simulink model "NMPC_UAV_MHE_CasaDi"  (R2022a)
settings: Solver=VariableStepAuto  StartTime=0.0  StopTime=60*2  RelTol=1e-3
values from neighbouring files (symbols this model uses):
  g = [g; st_next-st_next_RK4]    [MHE_CasaDi.m]    (also in UAVStateJacobianFcn.m = 9.81; UAV_parameters.m = 9.81)
  mass = 0.5    [MHE_CasaDi.m]    (also in UAV_parameters.m)
  Optitrack_Ts = 1/120    (= 0.00833333333333)    [Optitrack_parameters.m]
  Optitrack_var = [0.02e-3; 0.02e-3; 0.02e-3; 0.1*pi/180; 0.1*pi/180; 0.1*pi/180]    [Optitrack_parameters.m]
  Ts = 0.1    [MHE_CasaDi.m]    (also in UAV_parameters.m)
  XYThetaVPred = [1.99999737442 0.0050155230369 1.57305810416 0.100033273961 1.99990290242 0.0193669877756 1.58175256385 0.186831373139 1.99953586241 0.0406259992754 1.59458893555 0.23874169648 ... (4804 elements, 4x1201)]    [XYThetaVPred_wObstacles.mat]
  ZRef = 2*ones(1,60*2*10+1)    [UAV_parameters.m]
libraries: mpclib x1
settings Model: Creator=mrnel  LastModifiedBy=root

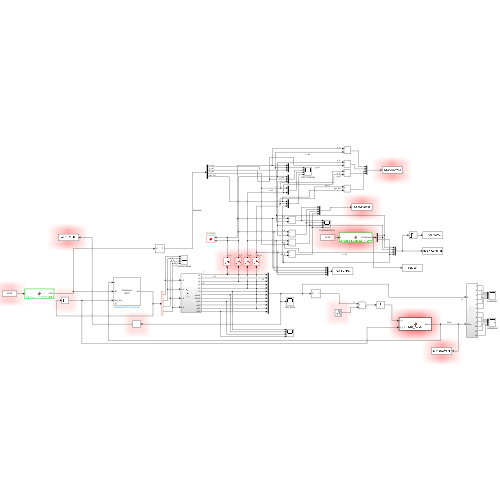
[thumbnail: Simulink's stored preview of the top-level diagram]
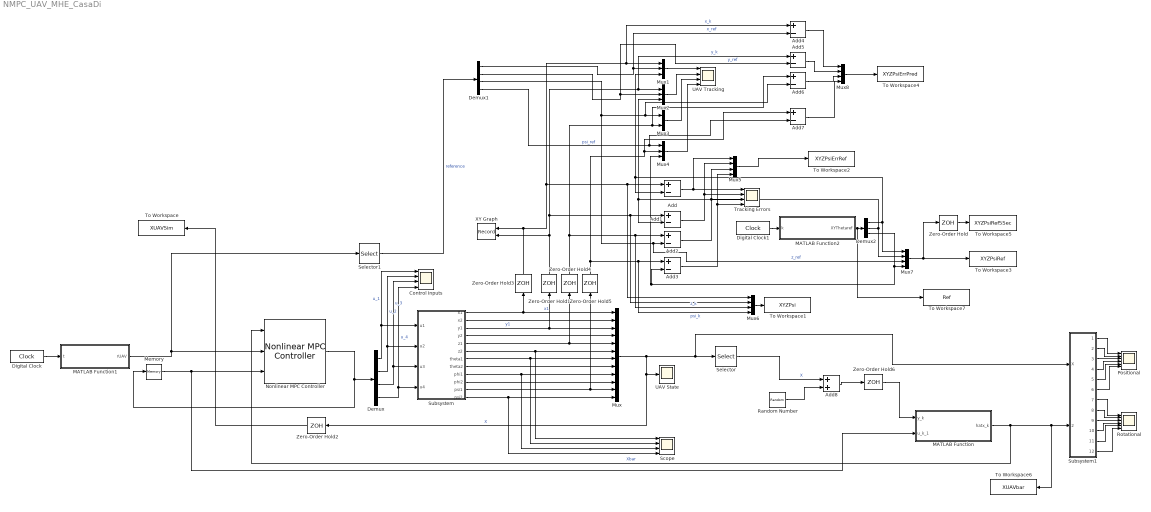
== system NMPC_UAV_MHE_CasaDi ==
  Add{,1..7} (8 alike) : Sum  Inputs=+-
  Add8 : Sum
  Control Inputs : Scope  NumInputPorts=4
  Demux : Demux
  Demux1 : Demux
  Demux2 : Demux  Outputs=3
  Digital Clock : DigitalClock  SampleTime=Ts
  Digital Clock1 : DigitalClock  SampleTime=Ts
  MATLAB Function : MATLAB Function  TreatAsAtomicUnit=on  SystemSampleTime=Ts
  MATLAB Function1 : MATLAB Function  TreatAsAtomicUnit=on
  MATLAB Function2 : MATLAB Function  TreatAsAtomicUnit=on  SystemSampleTime=Ts
  Memory : Memory  InitialCondition=[mass*g;0;0;0]  InheritSampleTime=on
  Mux : Mux  Inputs=12
  Mux1 : Mux  Inputs=3
  Mux2 : Mux  Inputs=3
  Mux3 : Mux  Inputs=2
  Mux4 : Mux  Inputs=3
  Mux{5..8} (4 alike) : Mux
  Nonlinear MPC Controller : mpclib/Nonlinear MPC Controller  nlmpcobj=nlmpcobj  UseObjectTs=on  UseMEX=off  md_enabled=off  mvtarget_enabled=off  param_enabled=off  cost_enabled=off  mvseq_enabled=off  stateseq_enabled=off  ovseq_enabled=off  slack_enabled=off  status_enabled=off  ov_min=off  ov_max=off  mv_min=off  mv_max=off  mvrate_min=off  mvrate_max=off  state_min=off  state_max=off  ov_weight=off  mv_weight=off  mvrate_weight=off  ecr_weight=off  nlp_initialize=off
  "Positional " : Scope  NumInputPorts=6
  Random Number : RandomNumber  Mean=zeros(6,1)  Variance=Optitrack_var.^2  SampleTime=Optitrack_Ts
  Rotational : Scope  NumInputPorts=6
  Scope : Scope  NumInputPorts=4
  Selector : Selector  NumberOfDimensions=2  InputPortWidth=3  IndexOptions=Index vector (dialog),Index vector (dialog)  Indices=[1 3 5 7 9 11],1  OutputSizes=1,1
  Selector1 : Selector  NumberOfDimensions=2  InputPortWidth=3  IndexOptions=Index vector (dialog),Index vector (dialog)  Indices=1,[1 3 5 11]  OutputSizes=1,1
  Subsystem : Subsystem
  Subsystem1 : Subsystem
  To Workspace : ToWorkspace  VariableName=XUAVSim  SaveFormat=Timeseries  SampleTime=Ts
  To Workspace1 : ToWorkspace  VariableName=XYZPsi  SaveFormat=Timeseries  SampleTime=0.1
  To Workspace2 : ToWorkspace  VariableName=XYZPsiErrRef  SaveFormat=Timeseries  SampleTime=Ts
  To Workspace3 : ToWorkspace  VariableName=XYZPsiRef  SaveFormat=Timeseries  SampleTime=0.1
  To Workspace4 : ToWorkspace  VariableName=XYZPsiErrPred  SaveFormat=Timeseries  SampleTime=Ts
  To Workspace5 : ToWorkspace  VariableName=XYZPsiRef5Sec  SaveFormat=Timeseries  SampleTime=5
  To Workspace6 : ToWorkspace  VariableName=XUAVbar  SaveFormat=Timeseries  SampleTime=Ts
  To Workspace7 : ToWorkspace  VariableName=Ref  SaveFormat=Timeseries  SampleTime=-1
  Tracking Errors : Scope  NumInputPorts=4
  UAV State : Scope
  UAV Tracking : Scope  NumInputPorts=4
  XY Graph : Record  FileSettingsInternal="{\"entries\":[{\"content\":{\"excelSettings\":{\"content\":{},\"type\":\"Streamout.ExcelSettings\"}},\"type\":\"Streamout.FileSettingStorage\",\"uuid\":\"\"}],\"packageUris\":[\"http:\\/\\/schema.mathworks.com\\/mf0\\/streamout_blocks\\/R2020a\"],\"version\":\"1.0\"}"  Layout=[1 1]  SignalsInternal="{\"entries\":[{\"content\":{\"signals\":[{\"content\":{\"blockPath\":[],\"channel\":[],\"dimensions\":[1],\"domain\":\"\",\"lineColor\":\"#a2142f\",\"plots\":[1],\"port\":1,\"sid\":[],\"signalID\":495,\"signalName\":\"x_k\"},\"type\":\"RecordBlkView.Signal\",\"uuid\":\"\"},{\"content\":{\"blockPath\":[],\"channel\":[],\"dimensions\":[1],\"domain\":\"\",\"lineColor\":\"#139fff\",\"plots\":[1],\"port\":2,\"sid\":[],\"signalID\":498,\"signalName\":\"y_k\"},\"type\":\"RecordBlkView.Signal\",\"uuid\":\"\"}]},\"type\":\"RecordBlkView.InputSignals\",\"uuid\":\"\"}],\"packageUris\":[\"http:\\/\\/schema.mathworks.com\\/mf0\\/streamout_blocks\\/R2020a\"],\"version\":\"1.0\"}"  VisualizationBindings="{\"xyplotplugin\":{\"info\":[{\"series\":[{\"bindingParametersList\":[{\"parameter\":\"X-Axis\",\"signalID\":495,\"signalName\":\"x_k\"},{\"parameter\":\"Y-Axis\",\"signalID\":498,\"signalName\":\"y_k\"}],\"seriesID\":20653}],\"subplotID\":1}]}}"  CompatibilityTag=XY
  Zero-Order Hold : ZeroOrderHold  SampleTime=5
  Zero-Order Hold{1..5} (5 alike) : ZeroOrderHold  SampleTime=Ts
  Zero-Order Hold6 : ZeroOrderHold  SampleTime=0.1
  wires:
  Demux/1 -> Control Inputs/1, Subsystem/1(u1)  "u_1"
  Demux/2 -> Control Inputs/2, Subsystem/2(u2)  "u_2"
  Nonlinear MPC Controller/1 -> Demux/1, Memory/1
  Subsystem/1(x1) -> Mux/1, Zero-Order Hold3/1  "x1"
  Subsystem/3(y1) -> Mux/3, Zero-Order Hold1/1  "y1"
  Zero-Order Hold2/1 -> To Workspace/1
  Digital Clock/1 -> MATLAB Function1/1(t)
  MATLAB Function1/1(rUAV) -> Nonlinear MPC Controller/2, Selector1/1
  Selector1/1 -> Demux1/1  "reference"
  Mux1/1 -> UAV Tracking/1
  Mux2/1 -> UAV Tracking/2
  Demux1/1 -> Add4/2, Mux1/2  "x_ref"
  Demux1/2 -> Mux2/2, Add5/2  "y_ref"
  Add/1 -> Mux5/1, Tracking Errors/1
  Add1/1 -> Mux5/2, Tracking Errors/2
  Mux5/1 -> To Workspace2/1
  Demux/3 -> Control Inputs/3, Subsystem/3(u3)  "u_3"
  Demux/4 -> Control Inputs/4, Subsystem/4(u4)  "u_4"
  Subsystem/2(x2) -> Mux/2
  Subsystem/4(y2) -> Mux/4
  Subsystem/5(z1) -> Zero-Order Hold4/1, Mux/5
  Subsystem/6(z2) -> Scope/1, Mux/6
  Subsystem/7(theta1) -> Scope/2, Mux/7
  Subsystem/8(theta2) -> Mux/8
  Subsystem/9(phi1) -> Scope/3, Mux/9
  Subsystem/10(phi2) -> Mux/10
  Subsystem/11(psi1) -> Mux/11, Zero-Order Hold5/1
  Subsystem/12(psi2) -> Scope/4, Mux/12
  Mux3/1 -> UAV Tracking/3
  Mux4/1 -> UAV Tracking/4
  Add2/1 -> Mux5/3, Tracking Errors/3
  Add3/1 -> Mux5/4, Tracking Errors/4
  Mux6/1 -> To Workspace1/1
  Digital Clock1/1 -> MATLAB Function2/1(k)
  MATLAB Function2/1(XYThetaref) -> To Workspace7/1, Demux2/1
  Demux2/2 -> Mux7/2, Add1/2, Mux2/3
  Demux2/1 -> Mux7/1, Mux1/3, Add/2
  Mux7/1 -> Zero-Order Hold/1, To Workspace3/1
  Demux1/3 -> Mux7/3, Add2/2, Add6/2, Mux3/1  "z_ref"
  Zero-Order Hold3/1 -> Mux6/1, Add/1, Add4/1, Mux1/1, XY Graph/1  "x_k"
  Demux1/4 -> Add7/2, Mux4/1  "psi_ref"
  Zero-Order Hold1/1 -> Mux6/2, Add1/1, Add5/1, Mux2/1, XY Graph/2  "y_k"
  Zero-Order Hold5/1 -> Add7/1, Mux4/2, Mux6/4, Add3/1  "psi_k"
  Zero-Order Hold4/1 -> Add6/1, Mux3/2, Mux6/3, Add2/1  "z_k"
  Mux8/1 -> To Workspace4/1
  Add4/1 -> Mux8/1
  Add5/1 -> Mux8/2
  Add6/1 -> Mux8/3
  Add7/1 -> Mux8/4
  Zero-Order Hold/1 -> To Workspace5/1
  Selector/1 -> Add8/1  "X"
  Add8/1 -> Zero-Order Hold6/1
  Random Number/1 -> Add8/2
  Zero-Order Hold6/1 -> MATLAB Function/1(y_k)
  Memory/1 -> MATLAB Function/2(u_k_1), Nonlinear MPC Controller/3
  MATLAB Function/1(hatx_k) -> Nonlinear MPC Controller/1, To Workspace6/1, Subsystem1/2(Xbar)  "Xbar"
  Subsystem1/9(Outport8) -> Rotational/3
  Subsystem1/11(Outport10) -> Rotational/5
  Subsystem1/4(Outport3) -> "Positional "/4
  Subsystem1/10(Outport9) -> Rotational/4
  Subsystem1/7(Outport6) -> Rotational/1
  Subsystem1/2(Outport1) -> "Positional "/2
  Subsystem1/1(Outport) -> "Positional "/1
  Subsystem1/5(Outport4) -> "Positional "/5
  Subsystem1/6(Outport5) -> "Positional "/6
  Subsystem1/12(Outport11) -> Rotational/6
  Mux/1 -> Subsystem1/1(X), Selector/1, UAV State/1, Zero-Order Hold2/1  "X"
  Subsystem1/3(Outport2) -> "Positional "/3
  Subsystem1/8(Outport7) -> Rotational/2
  Demux2/3 -> Mux4/3, Add3/2, Mux7/4

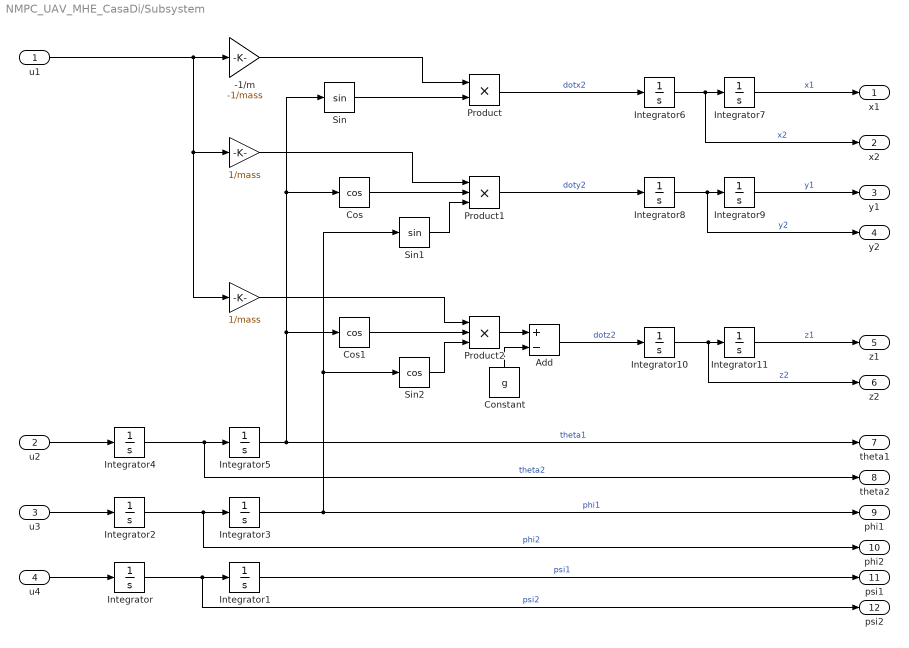
== system NMPC_UAV_MHE_CasaDi/Subsystem ==
  u1 : Inport
  u2 : Inport  Port=2
  u3 : Inport  Port=3
  u4 : Inport  Port=4
  " " : Gain  Gain=1/mass
  "  " : Gain  Gain=1/mass
  -1/m : Gain  Gain=-1/mass
  Add : Sum  Inputs=+-
  Constant : Constant  Value=g
  Cos : Trigonometry  Operator=cos
  Cos1 : Trigonometry  Operator=cos
  Integrator : Integrator  LimitOutput=on  UpperSaturationLimit=100*pi/180  LowerSaturationLimit=-100*pi/180
  Integrator1 : Integrator  InitialCondition=pi/2
  Integrator10 : Integrator  LimitOutput=on  UpperSaturationLimit=1  LowerSaturationLimit=-1
  Integrator11 : Integrator  InitialCondition=1  LimitOutput=on  LowerSaturationLimit=0
  Integrator{2,4,6,8..9} (5 alike) : Integrator
  Integrator3 : Integrator  LimitOutput=on  UpperSaturationLimit=30*pi/180  LowerSaturationLimit=-30*pi/180
  Integrator5 : Integrator  LimitOutput=on  UpperSaturationLimit=30*pi/180  LowerSaturationLimit=-30*pi/180
  Integrator7 : Integrator  InitialCondition=2
  Product : Product
  Product1 : Product  Inputs=3
  Product2 : Product  Inputs=3
  Sin : Trigonometry
  Sin1 : Trigonometry
  Sin2 : Trigonometry  Operator=cos
  x1 : Outport
  x2 : Outport  Port=2
  y1 : Outport  Port=3
  y2 : Outport  Port=4
  z1 : Outport  Port=5
  z2 : Outport  Port=6
  theta1 : Outport  Port=7
  theta2 : Outport  Port=8
  phi1 : Outport  Port=9
  phi2 : Outport  Port=10
  psi1 : Outport  Port=11
  psi2 : Outport  Port=12
  wires:
  Integrator7/1 -> x1/1  "x1"
  Integrator/1 -> psi2/1, Integrator1/1  "psi2"
  Sin2/1 -> Product2/3
  Integrator3/1 -> phi1/1, Sin2/1, Sin1/1  "phi1"
  u4/1 -> Integrator/1
  Cos/1 -> Product1/2
  Product1/1 -> Integrator8/1  "doty2"
  Product/1 -> Integrator6/1  "dotx2"
  u1/1 -> " "/1, "  "/1, -1/m/1
  Sin1/1 -> Product1/3
  Integrator2/1 -> phi2/1, Integrator3/1  "phi2"
  Integrator1/1 -> psi1/1  "psi1"
  "  "/1 -> Product1/1
  Product2/1 -> Add/1
  Sin/1 -> Product/2
  Integrator4/1 -> theta2/1, Integrator5/1  "theta2"
  Cos1/1 -> Product2/2
  " "/1 -> Product2/1
  Integrator6/1 -> x2/1, Integrator7/1  "x2"
  Integrator8/1 -> y2/1, Integrator9/1  "y2"
  -1/m/1 -> Product/1
  Integrator5/1 -> theta1/1, Cos1/1, Cos/1, Sin/1  "theta1"
  Integrator10/1 -> z2/1, Integrator11/1  "z2"
  Add/1 -> Integrator10/1  "dotz2"
  Constant/1 -> Add/2
  u3/1 -> Integrator2/1
  u2/1 -> Integrator4/1
  Integrator9/1 -> y1/1  "y1"
  Integrator11/1 -> z1/1  "z1"

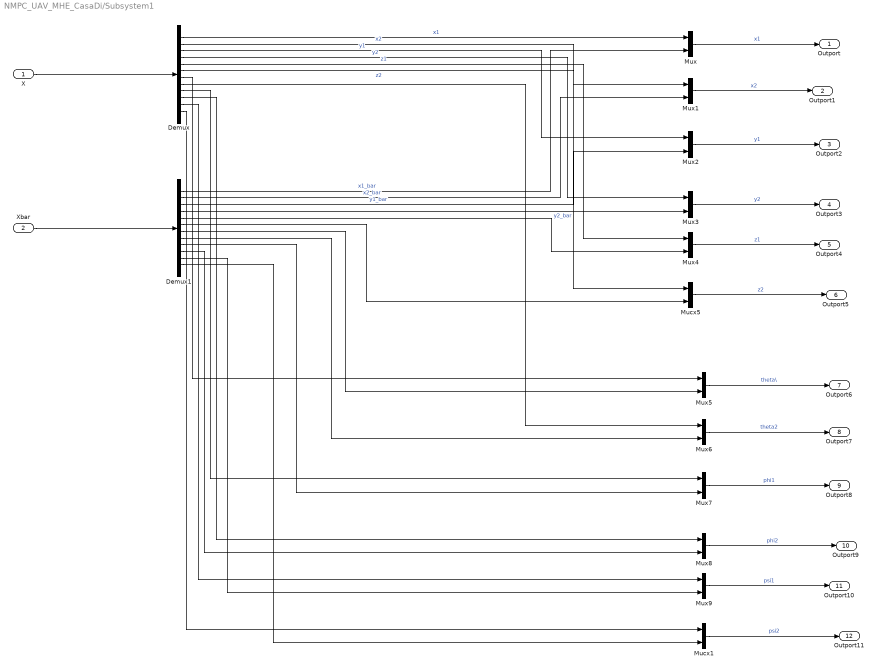
== system NMPC_UAV_MHE_CasaDi/Subsystem1 ==
  X : Inport
  Xbar : Inport  Port=2
  Demux : Demux  Outputs=12
  Demux1 : Demux  Outputs=12
  Mucx1 : Mux  Inputs=2
  Mucx5 : Mux  Inputs=2
  Mux{,1..9} (10 alike) : Mux  Inputs=2
  Outport : Outport
  Outport1 : Outport  Port=2
  Outport2 : Outport  Port=3
  Outport3 : Outport  Port=4
  Outport4 : Outport  Port=5
  Outport5 : Outport  Port=6
  Outport6 : Outport  Port=7
  Outport7 : Outport  Port=8
  Outport8 : Outport  Port=9
  Outport9 : Outport  Port=10
  Outport10 : Outport  Port=11
  Outport11 : Outport  Port=12
  wires:
  Demux1/1 -> Mux/2  "x1_bar"
  Demux1/3 -> Mux2/2  "y1_bar"
  Demux/11 -> Mux9/1
  Demux1/6 -> Mucx5/2
  Demux1/5 -> Mux4/2
  Demux1/2 -> Mux1/2  "x2_bar"
  Demux1/12 -> Mucx1/2
  Demux1/11 -> Mux9/2
  Demux1/4 -> Mux3/2  "y2_bar"
  Demux1/9 -> Mux7/2
  Demux/6 -> Mucx5/1  "z2"
  Demux/9 -> Mux7/1
  Demux1/7 -> Mux5/2
  Xbar/1 -> Demux1/1
  Demux/10 -> Mux8/1
  Demux/4 -> Mux3/1  "y2"
  Demux/7 -> Mux5/1
  Demux/5 -> Mux4/1  "z1"
  Demux/12 -> Mucx1/1
  Demux1/8 -> Mux6/2
  Demux/8 -> Mux6/1
  Demux/3 -> Mux2/1  "y1"
  Demux/1 -> Mux/1  "x1"
  Demux/2 -> Mux1/1  "x2"
  Demux1/10 -> Mux8/2
  X/1 -> Demux/1
  Mux/1 -> Outport/1  "x1"
  Mux1/1 -> Outport1/1  "x2"
  Mux2/1 -> Outport2/1  "y1"
  Mux3/1 -> Outport3/1  "y2"
  Mux4/1 -> Outport4/1  "z1"
  Mucx5/1 -> Outport5/1  "z2"
  Mux5/1 -> Outport6/1  "theta\\"
  Mux6/1 -> Outport7/1  "theta2"
  Mux8/1 -> Outport9/1  "phi2"
  Mux7/1 -> Outport8/1  "phi1"
  Mux9/1 -> Outport10/1  "psi1"
  Mucx1/1 -> Outport11/1  "psi2"

== matlab function NMPC_UAV_MHE_CasaDi/MATLAB Function1 ==
  settings: updateMethod=DISCRETE  sampleTime=Ts
  data: rUAV output; t input; Ts parameter; XYThetaVPred parameter; ZRef parameter
function rUAV = Compute_Reference_rUAV(t, Ts, XYThetaVPred, ZRef)
%COMPUTE_REFERENCE_RUAV This function extracts the reference r_{UAV}(k)
%defined in (43) at the current discrete time index k. r_{UAV}(k) that is
%used in the NMPC formulation is composed by the predicted pose of the
%ground vehicle for the next instant k+1 (this has been computed in a
%separate simulation) and the time-variant reference for the altitude.
%-------------------------------------------------------------------------
%Input
% t: current time instant
% Ts : sample time
% XYThetaVPred : predicted pose of the ground vehicle for the next instant 
%k+1 for all k over the simulation horizon
% ZRef : referenze for the drone altitude over the entire simulation horizon
%Output
% rUAV : reference used by the MPC defined in (45)
%=========================================================================

% Compute the discrete-time index k startig from the current time t and the
% the sample time Ts
k = int32(t/Ts) + 1;

% N. of state variables
nx = 12; 

% Initialize with all zeros the reference
rUAV = zeros(1,nx);

% x(k+1|k)
rUAV(:,1) = XYThetaVPred(1,k);

% y(k+1|k)
rUAV(:,3) = XYThetaVPred(2,k);

% z_{1,Ref}(k)
rUAV(:,5) = ZRef(1,k);

% theta(k+1|k)
rUAV(:,11) = XYThetaVPred(3,k);

== matlab function NMPC_UAV_MHE_CasaDi/MATLAB Function2 ==
  settings: updateMethod=DISCRETE  sampleTime=Ts
  data: XYThetaref output; k input
function XYThetaref = Compute_Reference_rT_UAV(k)
%COMPUTE_REFERENCE_RT_UAV Extract the components of reference r_{T,UAV}(k)
% defined in (44) x_{Ref}(k), y_{Ref}(k), and theta_{Ref}(k) at instant k
%-------------------------------------------------------------------------
%Input
% k: discrete-time index
% Ref : referenze r_{T,UAV} over the entire simulation horizon
%Output
% XYThetaref : x_{Ref}(k), y_{Ref}(k), and theta_{Ref}(k) at instant k
%=========================================================================

% Initialize the memory with zeros
XYThetaref = zeros(1,3);

% Extract the actual values x_{Ref}(k), y_{Ref}(k), and theta_{Ref}(k)
% Circle
w = 2*pi/(60);
XYThetaref = [2*cos(k*w) 2*sin(k*w) w*k+(pi/2)];

== matlab function NMPC_UAV_MHE_CasaDi/MATLAB Function ==
  data: y_k input; hatx_k output; u_k_1 input
function hatx_k = MHE_CasaDi(y_k, u_k_1)
%MHE_CASADI This function calls the MHE function. In particular the IPOPT
% solver is used to solve the nonlinear optimization problem
%-------------------------------------------------------------------------
%Input
% y_k : measurement at the current instant
% u_k_1 : control input at the current instant
%Output
% hatx_k : estimated state at the current instant
%=========================================================================

% In order to call the 'MHE_RK_CasaDi' MATLAB function with the CasaDi 
% library functions calls.
coder.extrinsic("MHE_CasaDi");

% Number of state variables
n_states = 12;

% Number of measurement variables
n_measurements = 6;

% Number of control variables
n_controls = 4;

% Prediction horizon
N_MHE = 5;

% drone mass
mass = 0.5;%[kg]

% gravitational acceleration
g = 9.81;%[ms^{-2}]

% At each iteration of the MHE, we want to store the batch of previous
% measuments and control inputs and the previous iteration estimate (this
% last is used as initial guess for the IPOPT solver)
persistent y_measurements u_cl X0

% Initialization of persisten values with zeros apart for z1 and u1

if(isempty(y_measurements))
    y_measurements = zeros(n_measurements,N_MHE+1);
    % x1 = 2 m
    y_measurements(1,:) = 2;
    % z1 = 1 m
    y_measurements(3,:) = 1;
    % phi1 = pi/2
    y_measurements(6,:) = pi/2;
end

if(isempty(u_cl))
    % CasaDi wants just one parameter vector, hence added one shadow value 
    % (i.e., below not N_MHE but N_MHE+1) 
    u_cl = zeros(n_controls,N_MHE+1);
    % u1 = mass*g
    u_cl(1,:) = mass*g;
end

if(isempty(X0))
    % initialization of the states decision variables
    X0 = zeros(N_MHE+1,n_states); 
    % z1 = 1 m
    X0(:,5) = 1; 
    % x1 = 2 m
    X0(:,1) = 2;
    % phi1 = pi/2
    X0(:,11) = pi/2;
end


% add current measurement
y_measurements = [y_measurements(:,2:end) y_k];

% add current control input
u_cl = [u_cl(:,2:end-1) u_k_1 u_cl(:,end)];

% call MHE CasaDi function
X_sol = MHE_CasaDi(y_measurements,u_cl,X0);

% return the estimate of the current state
hatx_k = zeros(n_states,1);
hatx_k = X_sol(N_MHE+1,1:n_states)';

% shift for the next step
X0 = [X_sol(2:(N_MHE+1),1:n_states); X_sol((N_MHE+1),1:n_states)];

end
